simulink model "DC_Mach"  (Simulink 4.00)
settings: Solver=ode45  StartTime=0.0  StopTime=2  MaxStep=1e-4  MinStep=1e-5  RelTol=1e-3  AbsTol=1e-4
InitFcn:
  | powericon('psbinitsys',bdroot);
libraries: powerlib2 x3
settings Model: LastModifiedBy=ieao  SaveTime=off  SaveOutput=off  LimitDataPoints=off  Decimation=2  BlockReductionOpt=off

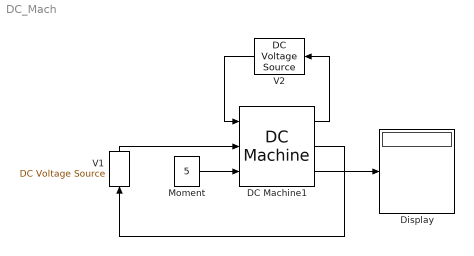
== system DC_Mach ==
  DC Machine1 : powerlib2/Machines/DC Machine  RLa="[ 2.52  0.048]"  RLf=[ 92 120]  Laf=0.207  J=0.01  Bm=0  Tf=0  w0=0  PSBOutputType=110
  Display : Display
      settings: Format=short  SampleTime=1e-3
  Moment : Constant  Value=5
  V1 : powerlib2/Electrical Sources/DC Voltage Source  Tag=PoWeRsYsTeMbLoCk  Description=source block  Orientation=up  V=220  mesure=None  PSBOutputType=1
  V2 : powerlib2/Electrical Sources/DC Voltage Source  Tag=PoWeRsYsTeMbLoCk  Description=source block  Orientation=left  V=220  mesure=None  PSBOutputType=1
  wires:
  V2/1 -> DC Machine1/1
  DC Machine1/1 -> V2/1
  DC Machine1/2 -> V1/1
  V1/1 -> DC Machine1/2
  DC Machine1/3 -> Display/1
  Moment/1 -> DC Machine1/3
